simulink model "SFCWTD_sim"  (R2016b)
settings: Solver=ode4  StartTime=0.0  StopTime=tend  FixedStep=0.001  RelTol=1e-3
values from neighbouring files (symbols this model uses):
  B = [1 0 0 0 0 0 0 0 0 0]    [10th.mat]
  D = [0.5 -0.2 0 0 0 0 0 0 0 0 -0.2 0.5 ... (100 elements, 10x10)]    [10th.mat]
  f = x(1:length(B))    [meuag.m]
  g = x(length(B)+1:2*length(B))    [meuag.m]
  K = [2 -1 0 0 0 0 0 0 0 0 -1 2 ... (100 elements, 10x10)]    [10th.mat]
  M = [1 0 0 0 0 0 0 0 0 0 0 1 ... (100 elements, 10x10)]    [10th.mat]
undefined symbols (not defined in the file or in its folder): tauf, taug, tauu, x0, xdot0
settings Model: Creator=danta  LastModifiedBy=danta

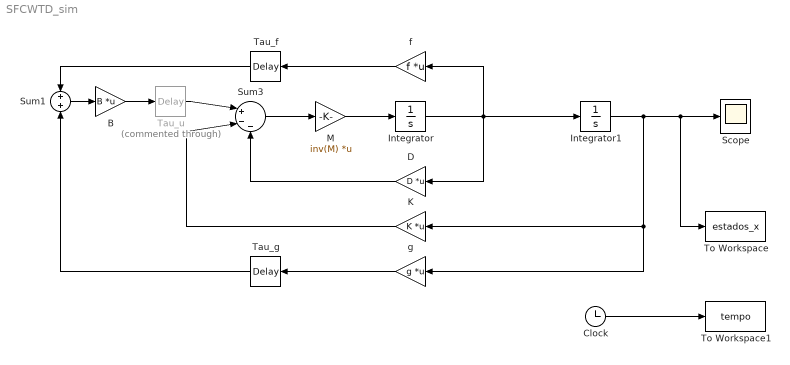
== system SFCWTD_sim ==
  B : Gain  Gain=B  Multiplication=Matrix(K*u)
  Clock : Clock
      settings: Decimation=tend
  D : Gain  Gain=D  Multiplication=Matrix(K*u)
  Integrator : Integrator  InitialCondition=xdot0
  Integrator1 : Integrator  InitialCondition=x0
  K : Gain  Gain=K  Multiplication=Matrix(K*u)
  M : Gain  Gain=inv(M)  Multiplication=Matrix(K*u)
  Scope : Scope
  Sum1 : Sum  Inputs=+|+
  Sum3 : Sum  Inputs=|+--
  Tau_f : TransportDelay  DelayTime=tauf
  Tau_g : TransportDelay  DelayTime=taug
  Tau_u : TransportDelay  Commented=through  DelayTime=tauu
  To Workspace : ToWorkspace  VariableName=estados_x  SampleTime=-1
  To Workspace1 : ToWorkspace  VariableName=tempo  SampleTime=-1
  f : Gain  Gain=f  Multiplication=Matrix(K*u)
  g : Gain  Gain=g  Multiplication=Matrix(K*u)
  wires:
  Sum3/1 -> M/1
  M/1 -> Integrator/1
  Integrator1/1 -> g/1, K/1, To Workspace/1, Scope/1
  Integrator/1 -> f/1, D/1, Integrator1/1
  D/1 -> Sum3/3
  K/1 -> Sum3/2
  Clock/1 -> To Workspace1/1
  g/1 -> Tau_g/1
  Tau_g/1 -> Sum1/2
  f/1 -> Tau_f/1
  Tau_f/1 -> Sum1/1
  Sum1/1 -> B/1
  B/1 -> Tau_u/1
  Tau_u/1 -> Sum3/1
